simulink model "rtwdemo_logicORsl"  (Simulink 7.1)
settings: Solver=FixedStepDiscrete  StartTime=0.0  StopTime=10.0  RelTol=1e-3
libraries: simulink x1
settings Model: Creator=ajayaram  LastModifiedBy=ajayaram
settings OptimizationCC: OptimizeModelRefInitCode=on  LifeSpan=1
settings RTWCC: SystemTargetFile=ert.tlc  GenCodeOnly=on  GenerateMakefile=off  TemplateMakefile=ert_default_tmf  Description=Real-Time Workshop Embedded Coder (no auto configuration)  GenerateReport=on  ProcessScript=ert_make_rtw_hook  IncludeHyperlinkInReport=on  LaunchReport=on
settings CodeAppCC: IgnoreCustomStorageClasses=off
settings ERTTargetCC: GenerateSampleERTMain=on  InlinedParameterPlacement=NonHierarchical  ERTCustomFileTemplate=example_file_process.tlc

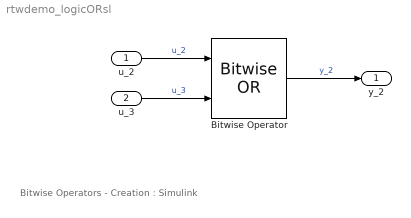
== system rtwdemo_logicORsl ==
  note: Bitwise Operators - Creation : Simulink
  u_2 : Inport  DataType=uint8  OutDataType=sfix(16)  OutScaling=2^0  OutDataTypeStr=uint8
  u_3 : Inport  Port=2  DataType=uint8  OutDataType=sfix(16)  OutScaling=2^0  OutDataTypeStr=uint8
  Bitwise Operator : simulink/Logic and Bit Operations/Bitwise Operator  logicop=OR  UseBitMask=off  NumInputPorts=2  BitMask=hex2dec('D8')  BitMaskRealWorld=Stored Integer
  y_2 : Outport  OutDataType=sfix(16)  OutScaling=2^0
  wires:
  Bitwise Operator/1 -> y_2/1  "y_2"
  u_2/1 -> Bitwise Operator/1  "u_2"
  u_3/1 -> Bitwise Operator/2  "u_3"
